simulink model "PowerSplitHEV_SpeedTracking"  (R2021a)
settings: Solver=daessc  StartTime=0.0  StopTime=t_end  RelTol=1e-3  AbsTol=1e-3  EnableMultiTasking=on
PreLoadFcn:
  | PowerSplitHEV_SpeedTracking_setup
libraries: fl_lib x1, nesl_utility x1
settings Model: FPTRunName=Active  PauseTimes=1397.4  SnapshotBufferSize=100  SnapshotInterval=100  Creator=MathWorks  LastModifiedBy=isaacito
settings SolverCC: AutoScaleAbsTol=off  DaesscMode=Fast  AlgebraicLoopSolver=TrustRegion
settings DataIOCC: LimitDataPoints=on  MaxDataPoints=15000  DSMLogging=off
settings OptimizationCC: ExpressionDepthLimit=2147483647  LifeSpan=inf
settings DebuggingCC: UnderspecifiedInitializationDetection=Classic  MergeDetectMultiDrivingBlocksExec=none  FcnCallInpInsideContextMsg=warning  StateNameClashWarn=warning  SFUnexpectedBacktrackingDiag=warning  SFNoUnconditionalDefaultTransitionDiag=warning  SFExecutionAtInitializationDiag=none  SFMachineParentedDataDiag=warning  ArithmeticOperatorsInVariantConditions=warning
settings HardwareCC: ProdBitPerPointer=32  ProdBitPerSizeT=32  ProdBitPerPtrDiffT=32  ProdLargestAtomicFloat=None  ProdIntDivRoundTo=Undefined  ProdEndianess=Unspecified  ProdWordSize=32  ProdHWDeviceType=32-bit Generic
settings ModelReferenceCC: PropagateSignalLabelsOutOfModel=off
settings SFSimCC: SimUseLocalCustomCode=off  CustomCodeUndefinedFunction=UseInterfaceOnly
settings RTWCC: RTWUseLocalCustomCode=off
settings CodeAppCC: StateflowObjectComments=on
settings GRTTargetCC: TargetLangStandard=C89/C90 (ANSI)  CombineOutputUpdateFcns=off  GRTInterface=on
settings ConfigComp: CovScope=Subsystem  CovMetricSettings=rw  CovEnableCumulative=off  CovSaveCumulativeToWorkspaceVar=on  CovSaveSingleToWorkspaceVar=on  CovExternalEMLEnable=off  CovSFcnEnable=off
settings SimscapeCC: SimscapeNominalValues="[{\"value\":\"20\",\"unit\":\"A\"},{\"value\":\"1\",\"unit\":\"bar\"},{\"value\":\"1\",\"unit\":\"cm^2\"},{\"value\":\"1\",\"unit\":\"cm^3/s\"},{\"value\":\"1\",\"unit\":\"kJ/kg\"},{\"value\":\"1\",\"unit\":\"kW\"},{\"value\":\"1\",\"unit\":\"l\"},{\"value\":\"1\",\"unit\":\"N\"},{\"value\":\"500\",\"unit\":\"N*m\"},{\"value\":\"1\",\"unit\":\"V\"}]"  SimscapeLogType=all  SimscapeLogSimulationStatistics=on  SimscapeLogName=logoutssc  SimscapeLogLimitData=off  SimscapeLogDataHistory=10000

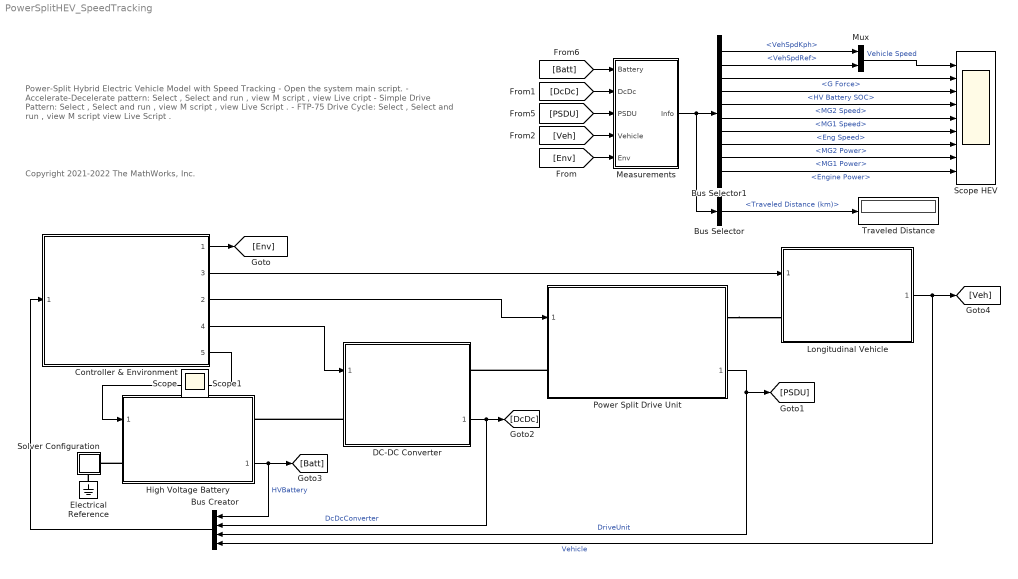
== system PowerSplitHEV_SpeedTracking ==
  note: Copyright 2021-2022 The MathWorks, Inc.
  note: Power-Split Hybrid Electric Vehicle Model with Speed Tracking
      | - Open the system main script.
      | - Accelerate-Decelerate pattern: Select , Select and run , view M script , view Live cript
      | - Simple Drive Pattern: Select , Select and run , view M script , view Live Script .
      | - FTP-75 Drive Cycle: Select , Select and run , view M script view Live Script .
  Bus Creator : BusCreator  Inputs=4
  Bus Selector : BusSelector  OutputSignals=Traveled Distance (km)
  Bus Selector1 : BusSelector  OutputSignals=VehSpdKph,VehSpdRef,G Force,HV Battery SOC,MG2 Speed,MG1 Speed,Eng Speed,MG2 Power,MG1 Power,Engine Power
  Controller & Environment : Subsystem  ReferencedSubsystem=PowerSplitHEV_SpeedTracking_DrvEnv_refsub
      settings: PortSchema="{\"entries\":[{\"content\":{\"sides\":[{\"content\":{\"connectorIds\":[\"In1\"]},\"type\":\"ConnectorPlacement.EquallySpacedRectSide\",\"uuid\":\"2556d520-c7d4-4516-9f86-304ff6f728f9\"},{\"content\":{\"connectorIds\":[\"Out1\",\"Out3\",\"Out2\",\"Out4\",\"Out5\"],\"side\":\"RIGHT\"},\"type\":\"ConnectorPlacement.EquallySpacedRectSide\",\"uuid\":\"062e0f2c-414b-4b92-aecb-aa366b4ba8cb\"},{\"content\":{\"connectorIds\":[],\"side\":\"TOP\"},\"type\":\"ConnectorPlacement.EquallySpacedRectSide\",\"uuid\":\"365a0e30-f0f0-4b3c-abb9-7309b547c7c1\"},{\"content\":{\"connectorIds\":[],\"side\":\"HIDDEN\"},\"type\":\"ConnectorPlacement.EquallySpacedRectSide\",\"uuid\":\"bc88ed38-4fcf-4515-9d3f-94734b03d6c8\"}]},\"type\":\"ConnectorPlacement.EquallySpacedConnector\",\"uuid\":\"e7d48425-03f4-4bdb-8b97-aad54198472d\"}],\"packageUris\":[\"http://schema.mathworks.com/mf0/Connector/R2020b\"],\"version\":\"1.0\"}"
  DC-DC Converter : Subsystem  ReferencedSubsystem=DcDcConverterElec_refsub
      settings: PortSchema="{\"entries\":[{\"content\":{\"sides\":[{\"content\":{\"connectorIds\":[\"In1\",\"LConn1\"]},\"type\":\"ConnectorPlacement.EquallySpacedRectSide\",\"uuid\":\"9fe8411b-04be-463e-9924-e5b159c802ea\"},{\"content\":{\"connectorIds\":[\"RConn1\",\"Out1\"],\"side\":\"RIGHT\"},\"type\":\"ConnectorPlacement.EquallySpacedRectSide\",\"uuid\":\"f74ab51b-f871-4eba-ad48-2355a260a50e\"},{\"content\":{\"connectorIds\":[],\"side\":\"TOP\"},\"type\":\"ConnectorPlacement.EquallySpacedRectSide\",\"uuid\":\"5fe4b190-e251-4a98-9e87-336539b68eba\"},{\"content\":{\"connectorIds\":[],\"side\":\"HIDDEN\"},\"type\":\"ConnectorPlacement.EquallySpacedRectSide\",\"uuid\":\"70e61028-3020-42d1-b1c6-53691d04cdd7\"}]},\"type\":\"ConnectorPlacement.EquallySpacedConnector\",\"uuid\":\"64b2eeb8-79e5-4be4-98bc-81a0cbd61baa\"}],\"packageUris\":[\"http://schema.mathworks.com/mf0/Connector/R2020b\"],\"version\":\"1.0\"}"
  Electrical Reference : fl_lib/Electrical/Electrical Elements/Electrical Reference
  High Voltage Battery : Subsystem  ReferencedSubsystem=BatteryHVElec_refsub
      settings: PortSchema="{\"entries\":[{\"content\":{\"sides\":[{\"content\":{\"connectorIds\":[\"In1\",\"LConn1\"]},\"type\":\"ConnectorPlacement.EquallySpacedRectSide\",\"uuid\":\"9fe8411b-04be-463e-9924-e5b159c802ea\"},{\"content\":{\"connectorIds\":[\"RConn1\",\"Out1\"],\"side\":\"RIGHT\"},\"type\":\"ConnectorPlacement.EquallySpacedRectSide\",\"uuid\":\"f74ab51b-f871-4eba-ad48-2355a260a50e\"},{\"content\":{\"connectorIds\":[],\"side\":\"TOP\"},\"type\":\"ConnectorPlacement.EquallySpacedRectSide\",\"uuid\":\"5fe4b190-e251-4a98-9e87-336539b68eba\"},{\"content\":{\"connectorIds\":[],\"side\":\"HIDDEN\"},\"type\":\"ConnectorPlacement.EquallySpacedRectSide\",\"uuid\":\"70e61028-3020-42d1-b1c6-53691d04cdd7\"}]},\"type\":\"ConnectorPlacement.EquallySpacedConnector\",\"uuid\":\"64b2eeb8-79e5-4be4-98bc-81a0cbd61baa\"}],\"packageUris\":[\"http://schema.mathworks.com/mf0/Connector/R2020b\"],\"version\":\"1.0\"}"
  Longitudinal Vehicle : Subsystem  ReferencedSubsystem=Vehicle1DBasic_refsub
  Measurements : Subsystem
  Mux : Mux  Inputs=2
  Power Split Drive Unit : Subsystem  ReferencedSubsystem=PowerSplitDriveUnitBasic_refsub
      settings: PortSchema="{\"entries\":[{\"content\":{\"sides\":[{\"content\":{\"connectorIds\":[\"In1\",\"LConn1\"]},\"type\":\"ConnectorPlacement.EquallySpacedRectSide\",\"uuid\":\"974aedaf-bb26-4d59-a293-409346043c39\"},{\"content\":{\"connectorIds\":[\"RConn1\",\"Out1\"],\"side\":\"RIGHT\"},\"type\":\"ConnectorPlacement.EquallySpacedRectSide\",\"uuid\":\"12ed2c12-3442-42d2-9925-d6af8f0a29b3\"},{\"content\":{\"connectorIds\":[],\"side\":\"TOP\"},\"type\":\"ConnectorPlacement.EquallySpacedRectSide\",\"uuid\":\"599325fb-3fa7-4117-9978-1ddfbbeb0247\"},{\"content\":{\"connectorIds\":[],\"side\":\"HIDDEN\"},\"type\":\"ConnectorPlacement.EquallySpacedRectSide\",\"uuid\":\"40453f65-ace7-4c7b-ae3d-0c837e197c38\"}]},\"type\":\"ConnectorPlacement.EquallySpacedConnector\",\"uuid\":\"841da484-ce2c-414e-826b-1cb66c55f7d7\"}],\"packageUris\":[\"http://schema.mathworks.com/mf0/Connector/R2020b\"],\"version\":\"1.0\"}"
  Scope HEV : Scope  NumInputPorts=9
  Solver Configuration : Subsystem
      settings: PortSchema="{\"entries\":[{\"content\":{\"sides\":[{\"content\":{\"connectorIds\":[]},\"type\":\"ConnectorPlacement.EquallySpacedRectSide\",\"uuid\":\"4a7e26c2-e9e9-4fea-b605-533b1a682be7\"},{\"content\":{\"connectorIds\":[\"RConn1\"],\"side\":\"RIGHT\"},\"type\":\"ConnectorPlacement.EquallySpacedRectSide\",\"uuid\":\"0210e324-555e-4372-b836-fcc8ab23e933\"},{\"content\":{\"connectorIds\":[],\"side\":\"TOP\"},\"type\":\"ConnectorPlacement.EquallySpacedRectSide\",\"uuid\":\"9bbae011-e6fc-4534-a44f-d79a5697c939\"},{\"content\":{\"connectorIds\":[\"RConn2\"],\"side\":\"BOTTOM\"},\"type\":\"ConnectorPlacement.EquallySpacedRectSide\",\"uuid\":\"d5829c0a-26ea-402d-a1c6-900997ddf1a8\"}]},\"type\":\"ConnectorPlacement.EquallySpacedConnector\",\"uuid\":\"f4e17c65-54c6-42fe-a467-9c6b014b697a\"}],\"packageUris\":[\"http://schema.mathworks.com/mf0/Connector/19700101\"],\"version\":\"1.0\"}"
  Traveled Distance : Display
  Scope : Scope
  Scope1 : Scope
  wires:
  [Batt] -> Measurements/1(Battery)
  Longitudinal Vehicle/1 -> Bus Creator/4, [Veh]  "Vehicle"
  [Env] -> Measurements/5(Env)
  Controller & Environment/3 -> Longitudinal Vehicle/1
  High Voltage Battery/1 -> [Batt], Bus Creator/1  "HVBattery"
  Controller & Environment/2 -> Power Split Drive Unit/1
  [Veh] -> Measurements/4(Vehicle)
  [PSDU] -> Measurements/3(PSDU)
  [DcDc] -> Measurements/2(DcDc)
  Bus Selector/1 -> Traveled Distance/1  "<Traveled Distance (km)>"
  Controller & Environment/1 -> [Env]
  Power Split Drive Unit/1 -> Bus Creator/3, [PSDU]  "DriveUnit"
  Bus Creator/1 -> Controller & Environment/1
  Measurements/1(Info) -> Bus Selector/1, Bus Selector1/1
  Bus Selector1/3 -> Scope HEV/2  "<G Force>"
  Bus Selector1/4 -> Scope HEV/3  "<HV Battery SOC>"
  Bus Selector1/5 -> Scope HEV/4  "<MG2 Speed>"
  Bus Selector1/6 -> Scope HEV/5  "<MG1 Speed>"
  Bus Selector1/7 -> Scope HEV/6  "<Eng Speed>"
  Mux/1 -> Scope HEV/1  "Vehicle Speed"
  Bus Selector1/1 -> Mux/1  "<VehSpdKph>"
  Bus Selector1/2 -> Mux/2  "<VehSpdRef>"
  Bus Selector1/8 -> Scope HEV/7  "<MG2 Power>"
  Bus Selector1/9 -> Scope HEV/8  "<MG1 Power>"
  Bus Selector1/10 -> Scope HEV/9  "<Engine Power>"
  DC-DC Converter/1 -> Bus Creator/2, [DcDc]  "DcDcConverter"
  Controller & Environment/4 -> DC-DC Converter/1
  Controller & Environment/5 -> High Voltage Battery/1
  connections:
  High Voltage Battery/LConn1 -- Solver Configuration/RConn1
  Electrical Reference/LConn1 -- Solver Configuration/RConn2
  DC-DC Converter/LConn1 -- High Voltage Battery/RConn1
  Power Split Drive Unit/LConn1 -- DC-DC Converter/RConn1
  Power Split Drive Unit/RConn1 -- Longitudinal Vehicle/LConn1

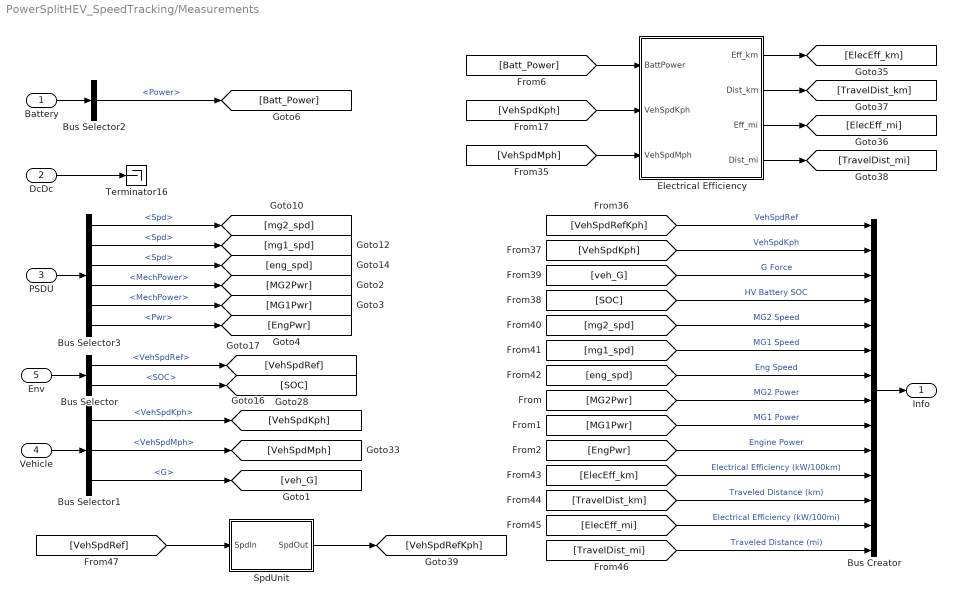
== system PowerSplitHEV_SpeedTracking/Measurements ==
  Battery : Inport
  DcDc : Inport  Port=2
  PSDU : Inport  Port=3
  Vehicle : Inport  Port=4
  Env : Inport  Port=5
  Bus Creator : BusCreator  Inputs=14
  Bus Selector : BusSelector  OutputSignals=VehSpdRef,SOC
  Bus Selector1 : BusSelector  OutputSignals=VehSpdKph,VehSpdMph,G
  Bus Selector2 : BusSelector  OutputSignals=Power
  Bus Selector3 : BusSelector  OutputSignals=mg2.Spd,mg1.Spd,eng.Spd,mg2.MechPower,mg1.MechPower,eng.Pwr
  Electrical Efficiency : Subsystem
  SpdUnit : Subsystem
  Terminator16 : Terminator
  Info : Outport
  wires:
  [Batt_Power] -> Electrical Efficiency/1(BattPower)
  [VehSpdKph] -> Electrical Efficiency/2(VehSpdKph)
  Env/1 -> Bus Selector/1
  Vehicle/1 -> Bus Selector1/1
  Bus Selector1/1 -> [VehSpdKph]  "<VehSpdKph>"
  Bus Selector1/3 -> [veh_G]  "<G>"
  Battery/1 -> Bus Selector2/1
  Bus Selector2/1 -> [Batt_Power]  "<Power>"
  PSDU/1 -> Bus Selector3/1
  Bus Selector3/1 -> [mg2_spd]  "<Spd>"
  Bus Selector3/2 -> [mg1_spd]  "<Spd>"
  Bus Selector3/3 -> [eng_spd]  "<Spd>"
  Bus Selector/1 -> [VehSpdRef]  "<VehSpdRef>"
  Bus Selector/2 -> [SOC]  "<SOC>"
  Bus Selector1/2 -> [VehSpdMph]  "<VehSpdMph>"
  [VehSpdMph] -> Electrical Efficiency/3(VehSpdMph)
  [VehSpdRefKph] -> Bus Creator/1  "VehSpdRef"
  [VehSpdKph] -> Bus Creator/2  "VehSpdKph"
  [veh_G] -> Bus Creator/3  "G Force"
  [SOC] -> Bus Creator/4  "HV Battery SOC"
  [mg2_spd] -> Bus Creator/5  "MG2 Speed"
  [mg1_spd] -> Bus Creator/6  "MG1 Speed"
  [eng_spd] -> Bus Creator/7  "Eng Speed"
  Electrical Efficiency/1(Eff_km) -> [ElecEff_km]
  Electrical Efficiency/3(Eff_mi) -> [ElecEff_mi]
  Electrical Efficiency/2(Dist_km) -> [TravelDist_km]
  Electrical Efficiency/4(Dist_mi) -> [TravelDist_mi]
  [ElecEff_km] -> Bus Creator/11  "Electrical Efficiency (kW/100km)"
  [TravelDist_km] -> Bus Creator/12  "Traveled Distance (km)"
  [ElecEff_mi] -> Bus Creator/13  "Electrical Efficiency (kW/100mi)"
  [TravelDist_mi] -> Bus Creator/14  "Traveled Distance (mi)"
  Bus Creator/1 -> Info/1
  [VehSpdRef] -> SpdUnit/1(SpdIn)
  SpdUnit/1(SpdOut) -> [VehSpdRefKph]
  Bus Selector3/4 -> [MG2Pwr]  "<MechPower>"
  Bus Selector3/5 -> [MG1Pwr]  "<MechPower>"
  Bus Selector3/6 -> [EngPwr]  "<Pwr>"
  [MG2Pwr] -> Bus Creator/8  "MG2 Power"
  [MG1Pwr] -> Bus Creator/9  "MG1 Power"
  [EngPwr] -> Bus Creator/10  "Engine Power"
  DcDc/1 -> Terminator16/1

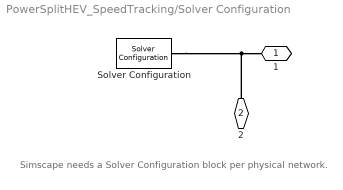
== system PowerSplitHEV_SpeedTracking/Solver Configuration ==
  note: Simscape needs a Solver Configuration block per physical network.
  Solver Configuration : nesl_utility/Solver Configuration  PhysicalDomain=network_engine_domain  SubClassName=solver  LeftPortType=input  RightPortType=generic  Tones=[]  Harmonics=[]  SimulateNoise=off  Profile=off  UseLocalSampling=off  EnableSwitchedLinearOptims=on  FrequencyDomain=off  UseCCode=off  RelTol=0.001  AbsTol=1e-06  MinStep=1e-09  ToWorkspace=off  RevertToSquareIcSolve=off  NumHomotopyIterations=100  PhasorMode=off  PhasorModeNumHarmonics=1  DoDC=off  ResidualTolerance=1e-9  UseLocalSolver=off  LocalSolverChoice=NE_BACKWARD_EULER_ADVANCER  LocalSolverSampleTime=0.01  DoFixedCost=off  MaxNonlinIter=3  MaxModeIter=2  ComputeImpulses=off  ImpulseIterations=2  LinearAlgebra=auto  EquationFormulation=NE_TIME_EF  DelaysMemoryBudget=1024  AutomaticFiltering=on  FilteringTimeConstant=0.001  PartitionStorageMethod=AS_NEEDED  PartitionMemoryBudget=1024  PartitionMethod=FAST
      settings: AttributesFormatString=Local solver %<UseLocalSolver>  SourceProductBaseCode=PW,SS
  1 : PMIOPort  Side=Right
  2 : PMIOPort  Port=2  Side=Right
  connections:
  Solver Configuration/RConn1 -- 1/RConn1 -- 2/RConn1

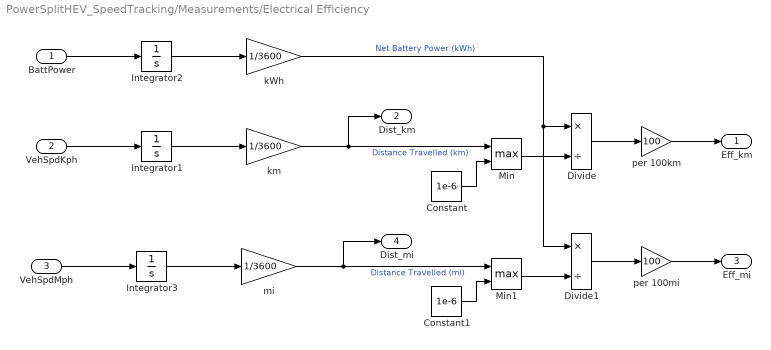
== system PowerSplitHEV_SpeedTracking/Measurements/Electrical Efficiency ==
  BattPower : Inport  Unit=kW
      settings: AttributesFormatString=%<Unit>
  VehSpdKph : Inport  Port=2  Unit=km/hr
      settings: AttributesFormatString=%<Unit>
  VehSpdMph : Inport  Port=3  Unit=mph
      settings: AttributesFormatString=%<Unit>
  Constant : Constant  Value=1e-6
  Constant1 : Constant  Value=1e-6
  Divide : Product  Inputs=*/
  Divide1 : Product  Inputs=*/
  Integrator1 : Integrator
      settings: AttributesFormatString=Initial Condition: %<InitialCondition>
  Integrator2 : Integrator
      settings: AttributesFormatString=Initial Condition: %<InitialCondition>
  Integrator3 : Integrator
      settings: AttributesFormatString=Initial Condition: %<InitialCondition>
  Min : MinMax  Function=max  Inputs=2
  Min1 : MinMax  Function=max  Inputs=2
  kWh : Gain  Gain=1/3600
  km : Gain  Gain=1/3600
  mi : Gain  Gain=1/3600
  per 100km : Gain  Gain=100
  per 100mi : Gain  Gain=100
  Eff_km : Outport
      settings: AttributesFormatString=%<Unit>
  Dist_km : Outport  Port=2  Unit=km
  Eff_mi : Outport  Port=3
      settings: AttributesFormatString=%<Unit>
  Dist_mi : Outport  Port=4  Unit=mi
  wires:
  per 100km/1 -> Eff_km/1
  Min/1 -> Divide/2
  Integrator1/1 -> km/1
  km/1 -> Dist_km/1, Min/1  "Distance Travelled (km)"
  Divide/1 -> per 100km/1
  Constant/1 -> Min/2
  kWh/1 -> Divide1/1, Divide/1  "Net Battery Power (kWh)"
  Integrator2/1 -> kWh/1
  BattPower/1 -> Integrator2/1
  VehSpdKph/1 -> Integrator1/1
  VehSpdMph/1 -> Integrator3/1
  Integrator3/1 -> mi/1
  per 100mi/1 -> Eff_mi/1
  Divide1/1 -> per 100mi/1
  Min1/1 -> Divide1/2
  mi/1 -> Dist_mi/1, Min1/1  "Distance Travelled (mi)"
  Constant1/1 -> Min1/2

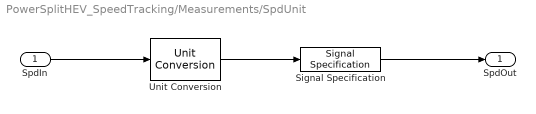
== system PowerSplitHEV_SpeedTracking/Measurements/SpdUnit ==
  SpdIn : Inport  Unit=m/s
      settings: AttributesFormatString=%<Unit>
  Signal Specification : SignalSpecification  Unit=km/hr
  Unit Conversion : UnitConversion
  SpdOut : Outport  Unit=km/hr
  wires:
  Unit Conversion/1 -> Signal Specification/1
  Signal Specification/1 -> SpdOut/1
  SpdIn/1 -> Unit Conversion/1
